simulink model "CONTROL_1R"  (R2019b)
settings: Solver=VariableStepAuto  StartTime=0.0  StopTime=1  RelTol=1e-3
undefined symbols (not defined in the file): d, fake_der, g, K, Kff, m, M, q0, qf, tau0, tau_max
libraries: simulink x1
settings Model: Creator=simone  LastModifiedBy=simone

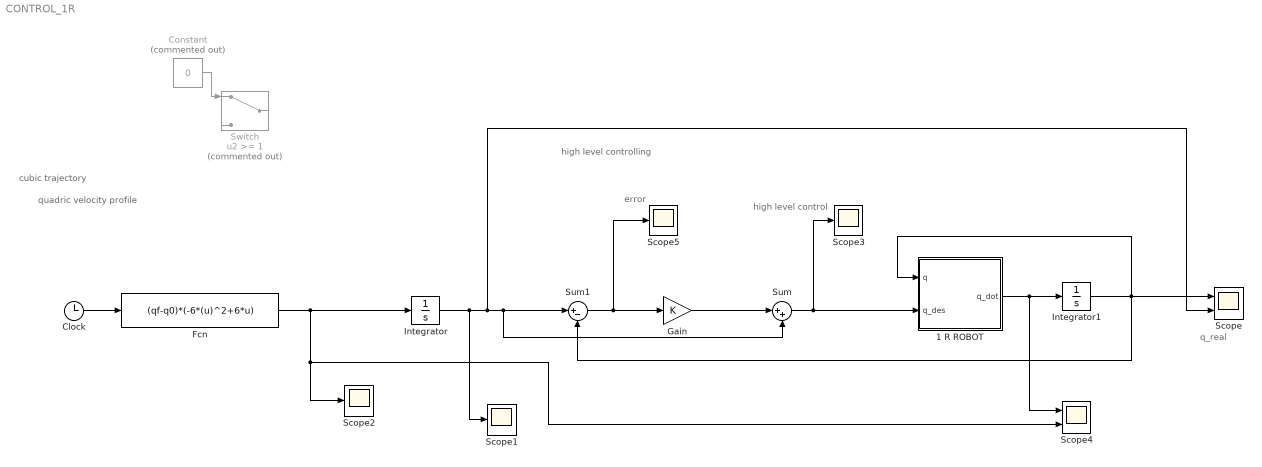
== system CONTROL_1R ==
  note: error
  note: high level controlling
  note: q_real
  note: high level control
  note: cubic trajectory
  note: quadric velocity profile
  1 R ROBOT : Subsystem
  Clock : Clock
  Constant : Constant  Commented=on  Value=0
  Fcn : Fcn  Expr=(qf-q0)*(-6*(u)^2+6*u)
  Gain : Gain  Gain=K
  Integrator : Integrator  InitialCondition=q0
  Integrator1 : Integrator  InitialCondition=q0
  Scope : Scope  NumInputPorts=2
  Scope{1..3,5} (4 alike) : Scope
  Scope4 : Scope  NumInputPorts=2
  Sum : Sum  Inputs=|++
  Sum1 : Sum  Inputs=|+-
  Switch : Switch  Commented=on  Threshold=1
  wires:
  Gain/1 -> Sum/1
  Sum/1 -> Scope3/1, 1 R ROBOT/2(q_des)
  1 R ROBOT/1(q_dot) -> Scope4/1, Integrator1/1
  Integrator/1 -> Scope/2, Sum1/1, Sum/2, Scope1/1
  Sum1/1 -> Scope5/1, Gain/1
  Integrator1/1 -> 1 R ROBOT/1(q), Scope/1, Sum1/2
  Constant/1 -> Switch/1
  Clock/1 -> Fcn/1
  Fcn/1 -> Integrator/1, Scope4/2, Scope2/1

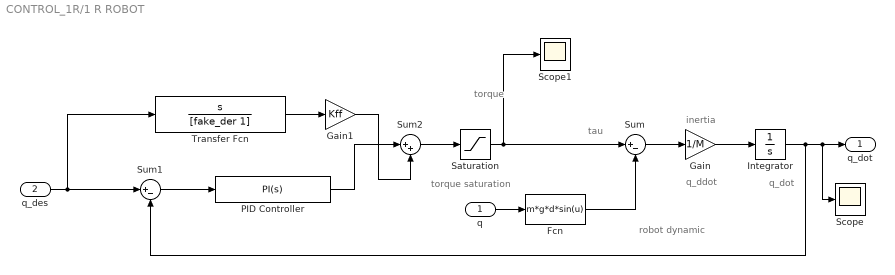
== system CONTROL_1R/1 R ROBOT ==
  note: torque saturation
  note: torque
  note: robot dynamic
  note: inertia
  note: q_ddot
  note: q_dot
  note: tau
  q : Inport
  q_des : Inport  Port=2
  Fcn : Fcn  Expr=m*g*d*sin(u)
  Gain : Gain  Gain=1/M
  Gain1 : Gain  Gain=Kff
  Integrator : Integrator  InitialCondition=tau0
  PID Controller : simulink/Continuous/PID Controller  Controller=PI  Form=Parallel  TimeDomain=Continuous-time  SampleTime=-1  IntegratorMethod=Forward Euler  FilterMethod=Forward Euler  ControllerParametersSource=internal  P=100  I=100  D=0  UseFilter=on  N=100  TunerSelectOption=Transfer Function Based (PID Tuner App)  InitialConditionSource=internal  InitialConditionForIntegrator=0  InitialConditionForFilter=0  DifferentiatorICPrevScaledInput=0  ExternalReset=none  TrackingMode=off  Kt=1  LimitOutput=off  UpperSaturationLimit=inf  LowerSaturationLimit=-inf  LinearizeAsGain=on  AntiWindupMode=none  Kb=1  POutMin=[]  POutMax=[]  IOutMin=[]  IOutMax=[]  DOutMin=[]  DOutMax=[]  NOutMin=[]  NOutMax=[]  SumOutMin=[]  SumOutMax=[]  SaturationOutMin=[]  SaturationOutMax=[]  PParamMin=[]  PParamMax=[]  IParamMin=[]  IParamMax=[]  DParamMin=[]  DParamMax=[]  NParamMin=[]  NParamMax=[]  KbParamMin=[]  KbParamMax=[]  KtParamMin=[]  KtParamMax=[]  KbOutMin=[]  KbOutMax=[]  KtOutMin=[]  KtOutMax=[]  IntegratorOutMin=[]  IntegratorOutMax=[]  FilterOutMin=[]  FilterOutMax=[]  SumI1OutMin=[]  SumI1OutMax=[]  SumI2OutMin=[]  SumI2OutMax=[]  SumI3OutMin=[]  SumI3OutMax=[]  SumI4OutMin=[]  SumI4OutMax=[]  SumDOutMin=[]  SumDOutMax=[]  DifferentiatorOutMin=[]  DifferentiatorOutMax=[]  FilterDiffOutCoefMin=[]  FilterDiffOutCoefMax=[]  ReciprocalOutMin=[]  ReciprocalOutMax=[]  SumDenOutMin=[]  SumDenOutMax=[]  SumNumOutMin=[]  SumNumOutMax=[]  DivideOutMin=[]  DivideOutMax=[]  IntegratorContinuousStateAttributes=''  IntegratorStateMustResolveToSignalObject=off  IntegratorRTWStateStorageClass=Auto  FilterContinuousStateAttributes=''  FilterStateMustResolveToSignalObject=off  FilterRTWStateStorageClass=Auto  ParallelPVariant=InternalParameters  IdealPVariant=Disabled  IVariant=InternalParameters  DVariant=Disabled  IntegratorVariant=Continuous  SatVariant=Disabled  AWVariant=Passthrough  PCopyVariant=Disabled  TRVariant=Disabled  FdbkBlocksVariant=Forward  IdealPFdbkVariant=Disabled  SatFdbkVariant=Disabled  DerivativeFilterVariant=Disabled  NVariant=Disabled  NCopyVariant=Disabled_SignalSpec  FilterICVariant=Disabled  IntegratorICVariant=InternalICs  ExternalResetVariant=Disabled  TRSumVariant=Passthrough  SumFdbkVariant=Disabled  SumVariant=Sum_PI
  Saturation : Saturate  UpperLimit=tau_max  LowerLimit=-tau_max
  Scope : Scope
  Scope1 : Scope
  Sum : Sum  Inputs=|+-
  Sum1 : Sum  Inputs=|+-
  Sum2 : Sum  Inputs=|++
  Transfer Fcn : TransferFcn  Numerator=[1 0]  Denominator=[fake_der 1]
  q_dot : Outport
  wires:
  PID Controller/1 -> Sum2/1
  Gain/1 -> Integrator/1
  Sum/1 -> Gain/1
  Gain1/1 -> Sum2/2
  Fcn/1 -> Sum/2
  q/1 -> Fcn/1
  Integrator/1 -> Scope/1, q_dot/1, Sum1/2
  q_des/1 -> Transfer Fcn/1, Sum1/1
  Transfer Fcn/1 -> Gain1/1
  Sum2/1 -> Saturation/1
  Saturation/1 -> Scope1/1, Sum/1
  Sum1/1 -> PID Controller/1
